simulink model "nonsim"  (Simulink 3.00)
settings: Solver=ode45  StartTime=0.0  StopTime=150.0  RelTol=1e-3
values from neighbouring files (symbols this model uses):
  a = 1    [fig3_18.m]    (also in fig3_31.m; fig3_32a.m; fig3_32b.m = 0.5; fig3_32c.m = 0.5)
  den = [1 1 2]    [fIg4_29.m]    (also in fig2_12.m = [1 0 g/L]; fig3_01.m = [1 k]; fig3_02.m = [1 k]; fig3_18.m = [1 a])
  num = 1/(m*L^2)    (= 2)    [fig2_12.m]    (also in fig3_01.m = 1; fig3_02.m = 1; fig3_18.m = [a]; fig3_19.m = [2 1])
undefined symbols (not defined in the file or in its folder): df, N, nf, r

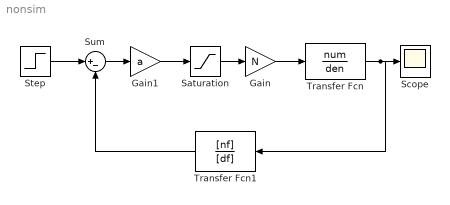
== system nonsim ==
  Gain : Gain  Gain=N  SaturateOnIntegerOverflow=on
  Gain1 : Gain  Gain=a  SaturateOnIntegerOverflow=on
  Saturation : Saturate  UpperLimit=1  LowerLimit=-1
  Scope : Scope
      settings: TimeRange=auto  YMin=-5  YMax=5  SaveName=yn  DataFormat=Matrix  LimitMaxRows=off
  Step : Step  Time=.1  Before=0  After=r  SampleTime=0.01
  Sum : Sum  Inputs=|+-  SaturateOnIntegerOverflow=on
  Transfer Fcn : TransferFcn  Numerator=num  Denominator=den
  Transfer Fcn1 : TransferFcn  Orientation=left  Numerator=[nf]  Denominator=[df]
  wires:
  Step/1 -> Sum/1
  Gain1/1 -> Saturation/1
  Sum/1 -> Gain1/1
  Saturation/1 -> Gain/1
  Gain/1 -> Transfer Fcn/1
  Transfer Fcn/1 -> Scope/1, Transfer Fcn1/1
  Transfer Fcn1/1 -> Sum/2
